simulink model "new_nncontroller_5_50"  (R2021a)
(part 13 of 14)

  "IW{5,4}(50,:)'" : Constant  Value=[-0.092260367604059201340760409948416054248809814453125;0.288608642474383725318176630025845952332019805908203125;-0.1792453026934868187680649498361162841320037841796875;0.065006810352411292797114583663642406463623046875;-0.08988995355681972387884570707683451473712921142578125;-0.688540255576554738325967264245264232158660888671875;-0.006265068906331716647173379897139966487884521484375;-0.77958545852877303428130062457057647407054901123046875;0.1901435522062191463277258662856183946132659912109375;0.7789840137625507754393083814647980034351348876953125;-0.9916466364493974339211490587331354618072509765625;-0.532596816006805529042367197689600288867950439453125;0.8789689466407535345382484592846594750881195068359375;-0.5765061058270897209609984201961196959018707275390625;0.1509575086333849736064394164714030921459197998046875;0.08054027966640120439478778280317783355712890625;-0.218163060752145643306221245438791811466217041015625;-0.6426299450798447221444575916393660008907318115234375;0.2008482148132293421127769761369563639163970947265625;0.617919961934332295783178778947331011295318603515625;-0.4549906952129527670791730997734703123569488525390625;0.82743688179984864472515937450225464999675750732421875;0.45914863598417365864179373602382838726043701171875;-0.5329757865584821008297922162455506622791290283203125;0.053784269916690462254305060696424334309995174407958984375;-0.649963135696746352465424934052862226963043212890625;-0.67707858355599037647465365807875059545040130615234375;-0.5671922358566929833756375955999828875064849853515625;0.62720964188067152011996086002909578382968902587890625;-0.78815444199557749271889406372793018817901611328125;0.702995240229719708935363087221048772335052490234375;0.1084728366433110602340406103394343517720699310302734375;-0.0203746450896591553558767628828718443401157855987548828125;0.0002487500444043888592204893939197063446044921875;-0.775653614720759332357147286529652774333953857421875;0.77724708196482350519573856217903085052967071533203125;-0.75369552011857887663381916354410350322723388671875;0.42678403822772015274722434696741402149200439453125;-0.550143658187712158991189426160417497158050537109375;0.88983770946706253202052039341651834547519683837890625;0.5398070204651970183107323464355431497097015380859375;-0.032331110427961183562128866242346703074872493743896484375;0.7234469323987393618580199472489766776561737060546875;-0.12498551862654243282957367000562953762710094451904296875;-0.7831262698633716379248426164849661290645599365234375;0.897910460826949918811124007334001362323760986328125;-0.899948092424768919528332844492979347705841064453125;0.8880315274086270083131466890336014330387115478515625;0.85420828567885698223705048803822137415409088134765625;0.70679731846291071750698620235198177397251129150390625]
      mask Display: e = 0.06;c1 = [120 150 230]/255;c2 = ([120 150 230]+0)/383;c3 = ([120 150 230]+128)/383;patch([0 1 1 0],[0 0 1 1],c1);patch([0 1 1 1-e 1-e 0+e],[0 0 1 1-e 0+e 0+e],c2);patch([0 0 1 1-e 0+e 0+e],[0 1 1 1-e 1-e 0+e],c3);plot([0 1 1 0 0],[0 0 1 1 0]);disp('weights');
  "IW{5,4}(6,:)'" : Constant  Value=[0.0145714096731367585835226208246240275911986827850341796875;-0.919767326024707454479312218609265983104705810546875;0.1025196579875821412120018294444889761507511138916015625;0.48495145634751590790756381466053426265716552734375;-0.91440491851849092785897710200515575706958770751953125;0.8184699961142707369532445227378048002719879150390625;-0.58093056540030030276966499513946473598480224609375;0.386300353609743518656927108168019913136959075927734375;-0.164525554281695907121729760547168552875518798828125;0.6898127664210720322301995111047290265560150146484375;0.62843803604852388478008151651010848581790924072265625;-0.219032678764314869823692788486368954181671142578125;-0.56429523655519542302272384404204785823822021484375;-0.50893603809006437987960680402466095983982086181640625;-0.360098756052208646138979020179249346256256103515625;-0.0298651878932745251660207941313274204730987548828125;-0.110026774580728403662988057476468384265899658203125;-0.81182574554892905638325828476808965206146240234375;0.372484263537190773973861723789013922214508056640625;0.86746021067575418417305854745791293680667877197265625;-0.6418165384645420079579025696148164570331573486328125;-0.6763835230542982746015923112281598150730133056640625;-0.871169278866029461738662575953640043735504150390625;0.5722255810135916664904698336613364517688751220703125;-0.321064600298221869412174100943957455456256866455078125;-0.9117207527185531290569997509010136127471923828125;-0.1356647084366936761856692328365170396864414215087890625;-0.170441854404427051150605620932765305042266845703125;0.9236678160836089279683847053092904388904571533203125;-0.9410458391343199391343432580470107495784759521484375;-0.035542563830460505158725936780683696269989013671875;0.38386853106450147254946614339132793247699737548828125;-0.69536288466720252987585126902558840811252593994140625;0.7758495173765631580664603461627848446369171142578125;-0.7662703898734226637401434345520101487636566162109375;0.6276547997014569890694701825850643217563629150390625;0.6133784332712248765773210834595374763011932373046875;-0.7823539668193018048469866698724217712879180908203125;-0.12554667758028126289815418203943409025669097900390625;0.069468369851627798094995114297489635646343231201171875;0.32319851522064890758656474645249545574188232421875;0.45782622198729827633911781958886422216892242431640625;-0.907193511436535704461903151241131126880645751953125;0.0504803820399725988732342329967650584876537322998046875;-0.09684422395902902991338123683817684650421142578125;-0.90523627962189312512464312021620571613311767578125;0.98976836153526637218647010740824043750762939453125;-0.1728739318401097957433876217692159116268157958984375;0.272634635616605114361021833246923051774501800537109375;-0.1043177191613685883542217425201670266687870025634765625]
      mask Display: e = 0.06;c1 = [120 150 230]/255;c2 = ([120 150 230]+0)/383;c3 = ([120 150 230]+128)/383;patch([0 1 1 0],[0 0 1 1],c1);patch([0 1 1 1-e 1-e 0+e],[0 0 1 1-e 0+e 0+e],c2);patch([0 0 1 1-e 0+e 0+e],[0 1 1 1-e 1-e 0+e],c3);plot([0 1 1 0 0],[0 0 1 1 0]);disp('weights');
  "IW{5,4}(7,:)'" : Constant  Value=[0.4093857125887534476049722798052243888378143310546875;0.028650611646671819698894978500902652740478515625;-0.104128180738226827628523096791468560695648193359375;0.786697394143356820706003418308682739734649658203125;0.753132839821508692779161719954572618007659912109375;-0.86488356131877974775079565006308257579803466796875;-0.77800034634235970543159055523574352264404296875;-0.1281350267269676379555676248855888843536376953125;0.5459592178287901997890685379388742148876190185546875;-0.047086715594744088519973956863395869731903076171875;-0.9877635934630626390884344800724647939205169677734375;-0.29653156832225846528672263957560062408447265625;-0.0216770415496714274894429763662628829479217529296875;0.227398296883349448904709788621403276920318603515625;0.22597791339003148181063806987367570400238037109375;0.506244531898635496958149815327487885951995849609375;-0.72075792316368136880555539391934871673583984375;-0.6270218532856397519736901813303120434284210205078125;-0.578165350294748581205794835113920271396636962890625;-0.7352371164877118392411148306564427912235260009765625;-0.4645665718075771000172835556440986692905426025390625;0.1408007431279838517212965598446317017078399658203125;-0.273715656078716396137906485819257795810699462890625;-0.904376228077623078860369787435047328472137451171875;-0.1007811462698315896346912268199957907199859619140625;0.007347121694520009071993627003394067287445068359375;0.3380433741269392999839737967704422771930694580078125;-0.2289760395420386007714341758401133120059967041015625;0.866356145325139603841080315760336816310882568359375;-0.333342813630977286010192983667366206645965576171875;0.416760901619977364163105448824353516101837158203125;-0.0048526531322024002435000511468388140201568603515625;0.604607335149959457254453809582628309726715087890625;0.874153803349613678363994040410034358501434326171875;0.55742074020402210265956455259583890438079833984375;-0.95964315049184190087316892459057271480560302734375;-0.457887469609615127552615376771427690982818603515625;0.91007910790181245630492412601597607135772705078125;-0.8547961159150847532117722948896698653697967529296875;-0.968259043291596288582923079957254230976104736328125;0.7202533065393306177526255851262249052524566650390625;-0.470364771532831849043532201903872191905975341796875;-0.5120560890633949480132969256374053657054901123046875;0.1444884561593593463868501203251071274280548095703125;0.489452838727210792768573810462839901447296142578125;-0.379657235532150583168231605668552219867706298828125;0.7569160897649658270580630414769984781742095947265625;-0.5806788258537329827646544799790717661380767822265625;0.6466885041343106710343136001029051840305328369140625;-0.9559857670299185539164454894489608705043792724609375]
      mask Display: e = 0.06;c1 = [120 150 230]/255;c2 = ([120 150 230]+0)/383;c3 = ([120 150 230]+128)/383;patch([0 1 1 0],[0 0 1 1],c1);patch([0 1 1 1-e 1-e 0+e],[0 0 1 1-e 0+e 0+e],c2);patch([0 0 1 1-e 0+e 0+e],[0 1 1 1-e 1-e 0+e],c3);plot([0 1 1 0 0],[0 0 1 1 0]);disp('weights');
  "IW{5,4}(8,:)'" : Constant  Value=[-0.2934138839856894609425808084779419004917144775390625;-0.9672759806646384905803870424279011785984039306640625;-0.2208996666821556598137021865113638341426849365234375;0.4288534632565863535802463957224972546100616455078125;0.51081944565320469564539962448179721832275390625;0.0216342503700375221598051211913116276264190673828125;0.0419286897745514419710843867505900561809539794921875;0.3415256187748665350767396375886164605617523193359375;0.27061306642126936594650032930076122283935546875;0.384111289781901898976457232492975890636444091796875;0.410856686526161585248928531655110418796539306640625;0.6841522366815964151243179003358818590641021728515625;0.2705688112448381144048425994697026908397674560546875;0.9806261502044504307917804908356629312038421630859375;-0.7486586960677861224411344664986245334148406982421875;-0.8148557074703430824769156970432959496974945068359375;0.8771554198332924823233724964666180312633514404296875;-0.6617929738627947866547174271545372903347015380859375;0.2689729671277298894693785769050009548664093017578125;-0.438348661888660284802199385012499988079071044921875;0.5493713820765926403311141257290728390216827392578125;-0.8553985398299064346616660259314812719821929931640625;-0.14530195868097894873471886967308819293975830078125;-0.93199366279616402408692010794766247272491455078125;0.17900169416811895217733763274736702442169189453125;0.0841054650854362595424618120887316763401031494140625;-0.1958958452406616146390661015175282955169677734375;0.69892062458842207917086852830834686756134033203125;0.269161626281525290238505476736463606357574462890625;-0.124732241451207759297403754317201673984527587890625;0.7145614052447151198776964520220644772052764892578125;-0.5367173183196740637868060730397701263427734375;-0.5327034558481908987914721365086734294891357421875;-0.4518355300879768332578123590792529284954071044921875;-0.0557733231011632302198677280102856457233428955078125;0.1930710543132871936933270262670703232288360595703125;0.861112360139955068660810866276733577251434326171875;-0.5913020579384526964616952682263217866420745849609375;-0.071394458633898150168306528939865529537200927734375;0.8032324459456299248216737396433018147945404052734375;0.8039951405369369918929578489041887223720550537109375;0.6550037458710364912661816561012528836727142333984375;-0.17115118995341749297267597285099327564239501953125;-0.7902769391491555328599361018859781324863433837890625;0.602571818332460207301437549176625907421112060546875;-0.6395640555997774701069147340604104101657867431640625;0.02932636553433365378396047162823379039764404296875;0.0140649879107963560187499751918949186801910400390625;-0.8175425299566170256326813614577986299991607666015625;-0.3897574962517413865725757204927504062652587890625]
      mask Display: e = 0.06;c1 = [120 150 230]/255;c2 = ([120 150 230]+0)/383;c3 = ([120 150 230]+128)/383;patch([0 1 1 0],[0 0 1 1],c1);patch([0 1 1 1-e 1-e 0+e],[0 0 1 1-e 0+e 0+e],c2);patch([0 0 1 1-e 0+e 0+e],[0 1 1 1-e 1-e 0+e],c3);plot([0 1 1 0 0],[0 0 1 1 0]);disp('weights');
  "IW{5,4}(9,:)'" : Constant  Value=[-0.825781956466138833405921104713343083858489990234375;-0.673671405949214818775772073422558605670928955078125;0.1784360557165054483874655488762073218822479248046875;-0.4906376117585649065944153335294686257839202880859375;0.302955945452832775544038668158464133739471435546875;-0.9806221138624990896204280943493358790874481201171875;0.2011161173845119609637777102761901915073394775390625;-0.8429039369132504955217655151500366628170013427734375;0.210928036609257407718587273848243057727813720703125;-0.24123591154488988053117282106541097164154052734375;-0.21191970748745614372410273062996566295623779296875;-0.5144540569513866845596794519224204123020172119140625;-0.862942123102181657401388292782939970493316650390625;-0.3212863875282032655178454660926945507526397705078125;-0.938650810002588542602097732014954090118408203125;0.1717815688716453070838952044141478836536407470703125;-0.130836063192326879089932845090515911579132080078125;-0.4696987850380660578508695834898389875888824462890625;-0.7033979310612921143075482177664525806903839111328125;0.619794580883736845322573572047986090183258056640625;0.10224030802002115336790666333399713039398193359375;-0.7029411327848078538949039284489117562770843505859375;-0.5495580802667083819557092283503152430057525634765625;-0.7315205747218447296376098165637813508510589599609375;0.3467736396358820361029984269407577812671661376953125;0.0033925438300002053182424788246862590312957763671875;0.5871042671155566328167196843423880636692047119140625;-0.420244364898484601411610128707252442836761474609375;0.9571650391778130373410249376320280134677886962890625;0.880659410507863782413551234640181064605712890625;0.5123406319780252626827632411732338368892669677734375;-0.2719743730191279684760274903965182602405548095703125;-0.6499531960519659978814388523460365831851959228515625;0.2187664157740669690355161947081796824932098388671875;0.712899544375499960580100378138013184070587158203125;-0.299716229877045936547119708848185837268829345703125;-0.1680234994926841363138692031498067080974578857421875;0.993420472620827776921714757918380200862884521484375;0.970798730673128051904541280237026512622833251953125;-0.513680835768670629448706677067093551158905029296875;-0.3749896502514078466816727086552418768405914306640625;-0.00488248477076158593490617931820452213287353515625;-0.9660935706428830371805815957486629486083984375;-0.6867350027306591275788605344132520258426666259765625;-0.071987549366349323776148594333790242671966552734375;-0.2438747537910541662853347588679753243923187255859375;-0.3662426598970129898447112282156012952327728271484375;0.436363597138454739621238331892527639865875244140625;0.577987736489344872126139307511039078235626220703125;-0.307300628334226555438135619624517858028411865234375]
      mask Display: e = 0.06;c1 = [120 150 230]/255;c2 = ([120 150 230]+0)/383;c3 = ([120 150 230]+128)/383;patch([0 1 1 0],[0 0 1 1],c1);patch([0 1 1 1-e 1-e 0+e],[0 0 1 1-e 0+e 0+e],c2);patch([0 0 1 1-e 0+e 0+e],[0 1 1 1-e 1-e 0+e],c3);plot([0 1 1 0 0],[0 0 1 1 0]);disp('weights');
  Mux : Mux  Inputs=50
      mask Display: e = 0.06;c1 = [120 150 230]/255;c2 = ([120 150 230]+0)/383;c3 = ([120 150 230]+128)/383;patch([0 1 1 0],[0 0 1 1],c1);patch([0 1 1 1-e 1-e 0+e],[0 0 1 1-e 0+e 0+e],c2);patch([0 0 1 1-e 0+e 0+e],[0 1 1 1-e 1-e 0+e],c3);plot([0 1 1 0 0],[0 0 1 1 0]);disp('Mux');
  dotprod{1..50} (50 alike) : neural/Weight Functions/dotprod
  "lz{5,4}" : Outport
      mask Display: e = 0.06;c1 = [120 230 180]/255;c2 = ([120 230 180]+0)/(256+128);c3 = ([120 230 180]+128)/(256+128);patch([0 1 1 0],[0 0 1 1],c1);patch([0 1 1 1-e 1-e 0+e],[0 0 1 1-e 0+e 0+e],c2);patch([0 0 1 1-e 0+e 0+e],[0 1 1 1-e 1-e 0+e],c3);plot([0 1 1 0 0],[0 0 1 1 0]);
  wires:
  "IW{5,4}(1,:)'"/1 -> dotprod1/1
  "ad{5,4}"/1 -> dotprod1/2, dotprod2/2, dotprod3/2, dotprod4/2, dotprod5/2, dotprod6/2, dotprod7/2, dotprod8/2, dotprod9/2, dotprod10/2, dotprod11/2, dotprod12/2, dotprod13/2, dotprod14/2, dotprod15/2, dotprod16/2, dotprod17/2, dotprod18/2, dotprod19/2, dotprod20/2, dotprod21/2, dotprod22/2, dotprod23/2, dotprod24/2, dotprod25/2, dotprod26/2, dotprod27/2, dotprod28/2, dotprod29/2, dotprod30/2, dotprod31/2, dotprod32/2, dotprod33/2, dotprod34/2, dotprod35/2, dotprod36/2, dotprod37/2, dotprod38/2, dotprod39/2, dotprod40/2, dotprod41/2, dotprod42/2, dotprod43/2, dotprod44/2, dotprod45/2, dotprod46/2, dotprod47/2, dotprod48/2, dotprod49/2, dotprod50/2
  dotprod1/1 -> Mux/1
  "IW{5,4}(2,:)'"/1 -> dotprod2/1
  dotprod2/1 -> Mux/2
  "IW{5,4}(3,:)'"/1 -> dotprod3/1
  dotprod3/1 -> Mux/3
  "IW{5,4}(4,:)'"/1 -> dotprod4/1
  dotprod4/1 -> Mux/4
  "IW{5,4}(5,:)'"/1 -> dotprod5/1
  dotprod5/1 -> Mux/5
  "IW{5,4}(6,:)'"/1 -> dotprod6/1
  dotprod6/1 -> Mux/6
  "IW{5,4}(7,:)'"/1 -> dotprod7/1
  dotprod7/1 -> Mux/7
  "IW{5,4}(8,:)'"/1 -> dotprod8/1
  dotprod8/1 -> Mux/8
  "IW{5,4}(9,:)'"/1 -> dotprod9/1
  dotprod9/1 -> Mux/9
  "IW{5,4}(10,:)'"/1 -> dotprod10/1
  dotprod10/1 -> Mux/10
  "IW{5,4}(11,:)'"/1 -> dotprod11/1
  dotprod11/1 -> Mux/11
  "IW{5,4}(12,:)'"/1 -> dotprod12/1
  dotprod12/1 -> Mux/12
  "IW{5,4}(13,:)'"/1 -> dotprod13/1
  dotprod13/1 -> Mux/13
  "IW{5,4}(14,:)'"/1 -> dotprod14/1
  dotprod14/1 -> Mux/14
  "IW{5,4}(15,:)'"/1 -> dotprod15/1
  dotprod15/1 -> Mux/15
  "IW{5,4}(16,:)'"/1 -> dotprod16/1
  dotprod16/1 -> Mux/16
  "IW{5,4}(17,:)'"/1 -> dotprod17/1
  dotprod17/1 -> Mux/17
  "IW{5,4}(18,:)'"/1 -> dotprod18/1
  dotprod18/1 -> Mux/18
  "IW{5,4}(19,:)'"/1 -> dotprod19/1
  dotprod19/1 -> Mux/19
  "IW{5,4}(20,:)'"/1 -> dotprod20/1
  dotprod20/1 -> Mux/20
  "IW{5,4}(21,:)'"/1 -> dotprod21/1
  dotprod21/1 -> Mux/21
  "IW{5,4}(22,:)'"/1 -> dotprod22/1
  dotprod22/1 -> Mux/22
  "IW{5,4}(23,:)'"/1 -> dotprod23/1
  dotprod23/1 -> Mux/23
  "IW{5,4}(24,:)'"/1 -> dotprod24/1
  dotprod24/1 -> Mux/24
  "IW{5,4}(25,:)'"/1 -> dotprod25/1
  dotprod25/1 -> Mux/25
  "IW{5,4}(26,:)'"/1 -> dotprod26/1
  dotprod26/1 -> Mux/26
  "IW{5,4}(27,:)'"/1 -> dotprod27/1
  dotprod27/1 -> Mux/27
  "IW{5,4}(28,:)'"/1 -> dotprod28/1
  dotprod28/1 -> Mux/28
  "IW{5,4}(29,:)'"/1 -> dotprod29/1
  dotprod29/1 -> Mux/29
  "IW{5,4}(30,:)'"/1 -> dotprod30/1
  dotprod30/1 -> Mux/30
  "IW{5,4}(31,:)'"/1 -> dotprod31/1
  dotprod31/1 -> Mux/31
  "IW{5,4}(32,:)'"/1 -> dotprod32/1
  dotprod32/1 -> Mux/32
  "IW{5,4}(33,:)'"/1 -> dotprod33/1
  dotprod33/1 -> Mux/33
  "IW{5,4}(34,:)'"/1 -> dotprod34/1
  dotprod34/1 -> Mux/34
  "IW{5,4}(35,:)'"/1 -> dotprod35/1
  dotprod35/1 -> Mux/35
  "IW{5,4}(36,:)'"/1 -> dotprod36/1
  dotprod36/1 -> Mux/36
  "IW{5,4}(37,:)'"/1 -> dotprod37/1
  dotprod37/1 -> Mux/37
  "IW{5,4}(38,:)'"/1 -> dotprod38/1
  dotprod38/1 -> Mux/38
  "IW{5,4}(39,:)'"/1 -> dotprod39/1
  dotprod39/1 -> Mux/39
  "IW{5,4}(40,:)'"/1 -> dotprod40/1
  dotprod40/1 -> Mux/40
  "IW{5,4}(41,:)'"/1 -> dotprod41/1
  dotprod41/1 -> Mux/41
  "IW{5,4}(42,:)'"/1 -> dotprod42/1
  dotprod42/1 -> Mux/42
  "IW{5,4}(43,:)'"/1 -> dotprod43/1
  dotprod43/1 -> Mux/43
  "IW{5,4}(44,:)'"/1 -> dotprod44/1
  dotprod44/1 -> Mux/44
  "IW{5,4}(45,:)'"/1 -> dotprod45/1
  dotprod45/1 -> Mux/45
  "IW{5,4}(46,:)'"/1 -> dotprod46/1
  dotprod46/1 -> Mux/46
  "IW{5,4}(47,:)'"/1 -> dotprod47/1
  dotprod47/1 -> Mux/47
  "IW{5,4}(48,:)'"/1 -> dotprod48/1
  dotprod48/1 -> Mux/48
  "IW{5,4}(49,:)'"/1 -> dotprod49/1
  dotprod49/1 -> Mux/49
  "IW{5,4}(50,:)'"/1 -> dotprod50/1
  dotprod50/1 -> Mux/50
  Mux/1 -> "lz{5,4}"/1
